simulink model "HeadlightManagement_Test_Harness"  (R2024a)
settings: Solver=FixedStepDiscrete  StartTime=0.0  StopTime=Inf  FixedStep=0.2  RelTol=1e-3  EnableMultiTasking=on
values from neighbouring files (symbols this model uses):
  Dem_EventStatusType : value not decoded    [dict.sldd]
undefined symbols (not defined in the file or in its folder): D1, P
libraries: simulink x6, autosarlibdem x2, autosarlibnvm x1
(part 2 of 2)

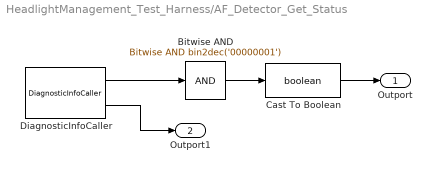
== system HeadlightManagement_Test_Harness/AF_Detector_Get_Status ==
  Bitwise AND : simulink/Logic and Bit Operations/Bitwise Operator  logicop=AND  UseBitMask=on  BitMask=bin2dec('00000001')  BitMaskRealWorld=Stored Integer
      settings: LibrarySourceBlock=|
      | simulink/Quick Insert/Logic and Bit
      | Operations/Bitwise AND
  Cast To Boolean : DataTypeConversion  OutDataTypeStr=boolean  SaturateOnIntegerOverflow=off  RndMeth=Floor
  DiagnosticInfoCaller : autosarlibdem/DiagnosticInfoCaller  PortName=AF_Detector  Operation=GetEventStatus  st=2  ServiceImpl=autosar.bsw.DemDiagnosticInfo  SyncToSchema=off
  Outport : Outport
  Outport1 : Outport  Port=2
  wires:
  Bitwise AND/1 -> Cast To Boolean/1
  Cast To Boolean/1 -> Outport/1
  DiagnosticInfoCaller/1 -> Bitwise AND/1
  DiagnosticInfoCaller/2 -> Outport1/1

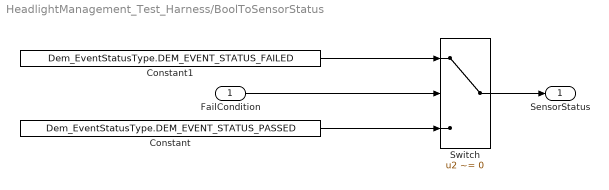
== system HeadlightManagement_Test_Harness/BoolToSensorStatus ==
  FailCondition : Inport
  Constant : Constant  Value=Dem_EventStatusType.DEM_EVENT_STATUS_PASSED
  Constant1 : Constant  Value=Dem_EventStatusType.DEM_EVENT_STATUS_FAILED
  Switch : Switch  Criteria=u2 ~= 0  SaturateOnIntegerOverflow=off  InputSameDT=off
  SensorStatus : Outport  VectorParamsAs1DForOutWhenUnconnected=off
  wires:
  FailCondition/1 -> Switch/2
  Constant/1 -> Switch/3
  Constant1/1 -> Switch/1
  Switch/1 -> SensorStatus/1

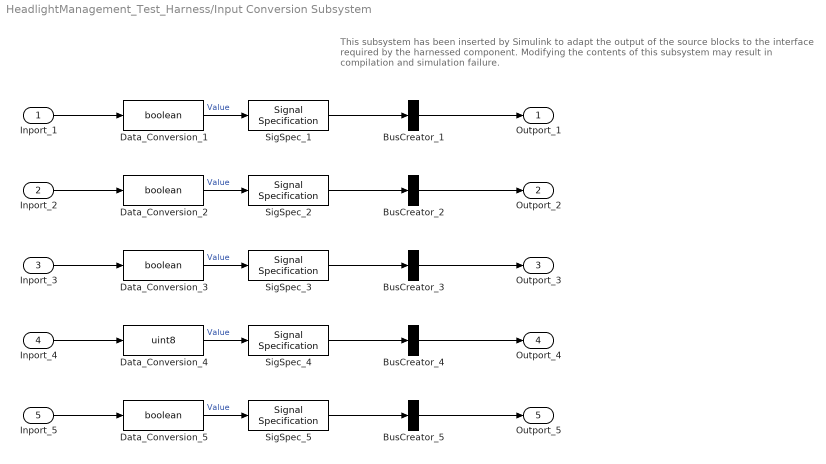
== system HeadlightManagement_Test_Harness/Input Conversion Subsystem ==
  note: This subsystem has been inserted by Simulink to adapt the output of the source blocks to the interface required by the harnessed component.
      |  Modifying the contents of this subsystem may result in compilation and simulation failure.
  Inport_1 : Inport
  Inport_2 : Inport  Port=2
  Inport_3 : Inport  Port=3
  Inport_4 : Inport  Port=4
  Inport_5 : Inport  Port=5
  BusCreator_1 : BusCreator  Inputs=1  OutDataTypeStr=Bus: Sensor_to_Ctrl
  BusCreator_2 : BusCreator  Inputs=1  OutDataTypeStr=Bus: Sensor_to_Ctrl
  BusCreator_3 : BusCreator  Inputs=1  OutDataTypeStr=Bus: HighBeam_Cmd
  BusCreator_4 : BusCreator  Inputs=1  OutDataTypeStr=Bus: TurnSignal_Cmd
  BusCreator_5 : BusCreator  Inputs=1  OutDataTypeStr=Bus: Ignition_State
  Data_Conversion_{1..3,5} (4 alike) : DataTypeConversion  OutDataTypeStr=boolean
  Data_Conversion_4 : DataTypeConversion  OutDataTypeStr=uint8
  SigSpec_1 : SignalSpecification  OutDataTypeStr=boolean  Dimensions=[1]  SampleTime=[-1, 0]
  SigSpec_2 : SignalSpecification  OutDataTypeStr=boolean  Dimensions=[1]  SampleTime=[-1, 0]
  SigSpec_3 : SignalSpecification  OutDataTypeStr=boolean  Dimensions=[1]  SampleTime=0.2
  SigSpec_4 : SignalSpecification  OutDataTypeStr=uint8  Dimensions=[1]  SampleTime=0.2
  SigSpec_5 : SignalSpecification  OutDataTypeStr=boolean  Dimensions=[1]  SampleTime=[-1, 0]
  Outport_1 : Outport
  Outport_2 : Outport  Port=2
  Outport_3 : Outport  Port=3
  Outport_4 : Outport  Port=4
  Outport_5 : Outport  Port=5
  wires:
  BusCreator_1/1 -> Outport_1/1
  SigSpec_1/1 -> BusCreator_1/1
  Data_Conversion_1/1 -> SigSpec_1/1  "Value"
  Inport_1/1 -> Data_Conversion_1/1
  BusCreator_2/1 -> Outport_2/1
  SigSpec_2/1 -> BusCreator_2/1
  Data_Conversion_2/1 -> SigSpec_2/1  "Value"
  Inport_2/1 -> Data_Conversion_2/1
  BusCreator_3/1 -> Outport_3/1
  SigSpec_3/1 -> BusCreator_3/1
  Data_Conversion_3/1 -> SigSpec_3/1  "Value"
  Inport_3/1 -> Data_Conversion_3/1
  BusCreator_4/1 -> Outport_4/1
  SigSpec_4/1 -> BusCreator_4/1
  Data_Conversion_4/1 -> SigSpec_4/1  "Value"
  Inport_4/1 -> Data_Conversion_4/1
  BusCreator_5/1 -> Outport_5/1
  SigSpec_5/1 -> BusCreator_5/1
  Data_Conversion_5/1 -> SigSpec_5/1  "Value"
  Inport_5/1 -> Data_Conversion_5/1

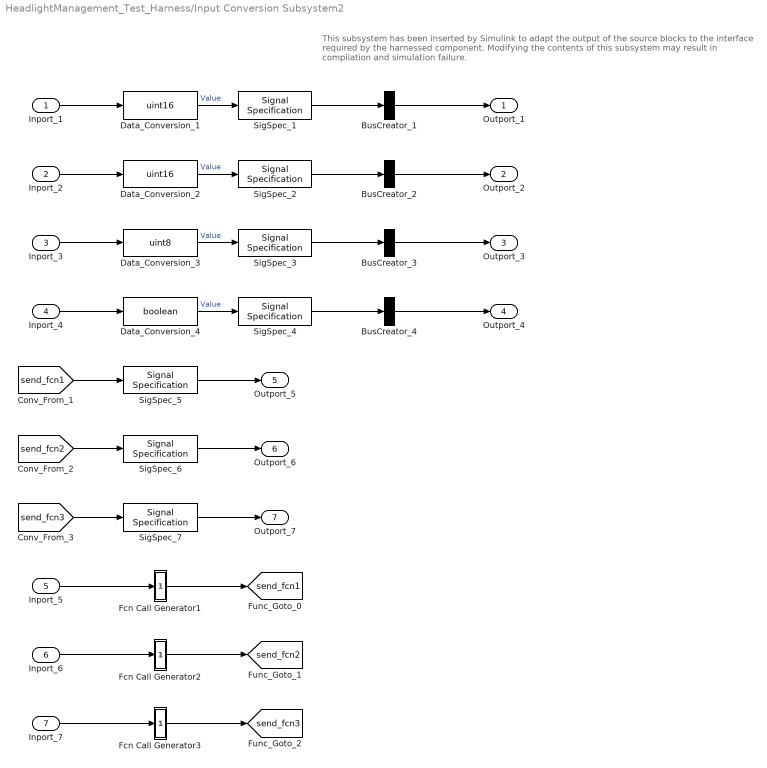
== system HeadlightManagement_Test_Harness/Input Conversion Subsystem2 ==
  note: This subsystem has been inserted by Simulink to adapt the output of the source blocks to the interface required by the harnessed component.
      |  Modifying the contents of this subsystem may result in compilation and simulation failure.
  Inport_1 : Inport
  Inport_2 : Inport  Port=2
  Inport_3 : Inport  Port=3
  Inport_4 : Inport  Port=4
  Inport_5 : Inport  Port=5
  Inport_6 : Inport  Port=6
  Inport_7 : Inport  Port=7
  BusCreator_1 : BusCreator  Inputs=1  OutDataTypeStr=Bus: Light_Data
  BusCreator_2 : BusCreator  Inputs=1  OutDataTypeStr=Bus: Visibility_Distance
  BusCreator_3 : BusCreator  Inputs=1  OutDataTypeStr=Bus: Humidity_Data
  BusCreator_4 : BusCreator  Inputs=1  OutDataTypeStr=Bus: Ignition_State
  Data_Conversion_1 : DataTypeConversion  OutDataTypeStr=uint16
  Data_Conversion_2 : DataTypeConversion  OutDataTypeStr=uint16
  Data_Conversion_3 : DataTypeConversion  OutDataTypeStr=uint8
  Data_Conversion_4 : DataTypeConversion  OutDataTypeStr=boolean
  Fcn Call Generator1 : Subsystem  Tag=_SLT_FCN_CALL_GEN_BLK_  mask(Function Call Generator Subsystem){sample_time=-1}
      mask prompts: sample_time "Sample time:"
      settings: LibrarySourceBlock=sltestutillib/fcn_call_gen
  Fcn Call Generator2 : Subsystem  Tag=_SLT_FCN_CALL_GEN_BLK_  mask(Function Call Generator Subsystem){sample_time=-1}
      mask prompts: sample_time "Sample time:"
      settings: LibrarySourceBlock=sltestutillib/fcn_call_gen
  Fcn Call Generator3 : Subsystem  Tag=_SLT_FCN_CALL_GEN_BLK_  mask(Function Call Generator Subsystem){sample_time=-1}
      mask prompts: sample_time "Sample time:"
      settings: LibrarySourceBlock=sltestutillib/fcn_call_gen
  SigSpec_1 : SignalSpecification  OutDataTypeStr=uint16  Unit=lx  Dimensions=[1]
  SigSpec_2 : SignalSpecification  OutDataTypeStr=uint16  Unit=meter  Dimensions=[1]
  SigSpec_3 : SignalSpecification  OutDataTypeStr=uint8  Unit=%RH  Dimensions=[1]
  SigSpec_4 : SignalSpecification  OutDataTypeStr=boolean  Dimensions=[1]
  SigSpec_5 : SignalSpecification
  SigSpec_6 : SignalSpecification
  SigSpec_7 : SignalSpecification
  Outport_1 : Outport
  Outport_2 : Outport  Port=2
  Outport_3 : Outport  Port=3
  Outport_4 : Outport  Port=4
  Outport_5 : Outport  Port=5
  Outport_6 : Outport  Port=6
  Outport_7 : Outport  Port=7
  tag scope: send_fcn1=global, send_fcn2=global, send_fcn3=global
  wires:
  BusCreator_1/1 -> Outport_1/1
  SigSpec_1/1 -> BusCreator_1/1
  Data_Conversion_1/1 -> SigSpec_1/1  "Value"
  Inport_1/1 -> Data_Conversion_1/1
  BusCreator_2/1 -> Outport_2/1
  SigSpec_2/1 -> BusCreator_2/1
  Data_Conversion_2/1 -> SigSpec_2/1  "Value"
  Inport_2/1 -> Data_Conversion_2/1
  BusCreator_3/1 -> Outport_3/1
  SigSpec_3/1 -> BusCreator_3/1
  Data_Conversion_3/1 -> SigSpec_3/1  "Value"
  Inport_3/1 -> Data_Conversion_3/1
  BusCreator_4/1 -> Outport_4/1
  SigSpec_4/1 -> BusCreator_4/1
  Data_Conversion_4/1 -> SigSpec_4/1  "Value"
  Inport_4/1 -> Data_Conversion_4/1
  SigSpec_5/1 -> Outport_5/1
  [send_fcn1] -> SigSpec_5/1
  SigSpec_6/1 -> Outport_6/1
  [send_fcn2] -> SigSpec_6/1
  SigSpec_7/1 -> Outport_7/1
  [send_fcn3] -> SigSpec_7/1
  Fcn Call Generator1/1(Out1) -> [send_fcn1]
  Inport_5/1 -> Fcn Call Generator1/1(In1)
  Fcn Call Generator2/1(Out1) -> [send_fcn2]
  Inport_6/1 -> Fcn Call Generator2/1(In1)
  Fcn Call Generator3/1(Out1) -> [send_fcn3]
  Inport_7/1 -> Fcn Call Generator3/1(In1)

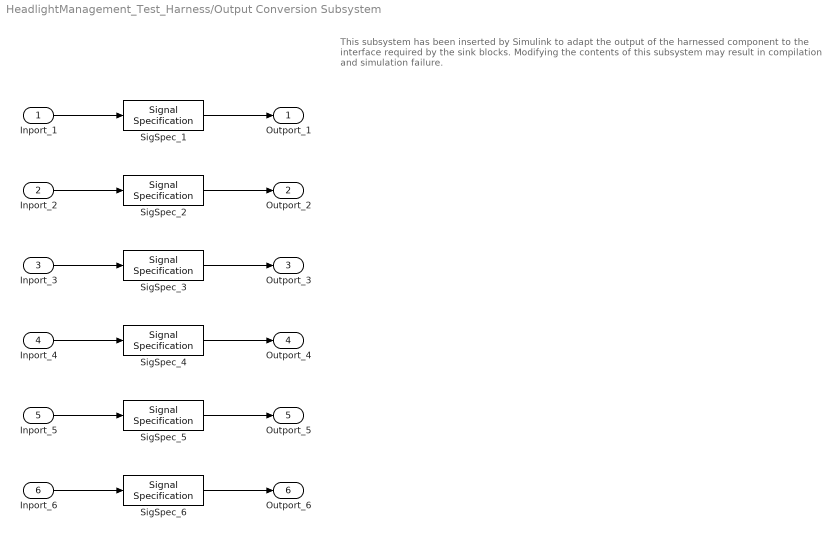
== system HeadlightManagement_Test_Harness/Output Conversion Subsystem ==
  note: This subsystem has been inserted by Simulink to adapt the output of the harnessed component to the interface required by the sink blocks.
      |  Modifying the contents of this subsystem may result in compilation and simulation failure.
  Inport_1 : Inport
  Inport_2 : Inport  Port=2
  Inport_3 : Inport  Port=3
  Inport_4 : Inport  Port=4
  Inport_5 : Inport  Port=5
  Inport_6 : Inport  Port=6
  SigSpec_{1..6} (6 alike) : SignalSpecification  Dimensions=[-1]  SampleTime=0.2
  Outport_1 : Outport
  Outport_2 : Outport  Port=2
  Outport_3 : Outport  Port=3
  Outport_4 : Outport  Port=4
  Outport_5 : Outport  Port=5
  Outport_6 : Outport  Port=6
  wires:
  Inport_1/1 -> SigSpec_1/1
  SigSpec_1/1 -> Outport_1/1
  Inport_2/1 -> SigSpec_2/1
  SigSpec_2/1 -> Outport_2/1
  Inport_3/1 -> SigSpec_3/1
  SigSpec_3/1 -> Outport_3/1
  Inport_4/1 -> SigSpec_4/1
  SigSpec_4/1 -> Outport_4/1
  Inport_5/1 -> SigSpec_5/1
  SigSpec_5/1 -> Outport_5/1
  Inport_6/1 -> SigSpec_6/1
  SigSpec_6/1 -> Outport_6/1

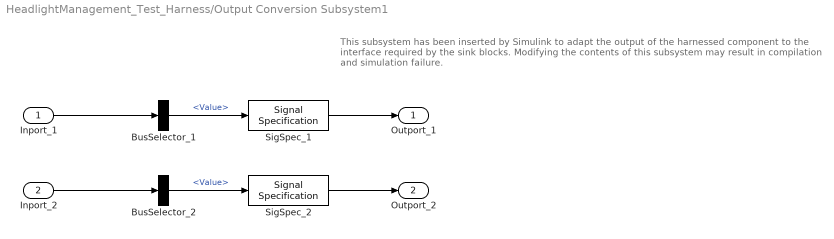
== system HeadlightManagement_Test_Harness/Output Conversion Subsystem1 ==
  note: This subsystem has been inserted by Simulink to adapt the output of the harnessed component to the interface required by the sink blocks.
      |  Modifying the contents of this subsystem may result in compilation and simulation failure.
  Inport_1 : Inport
  Inport_2 : Inport  Port=2
  BusSelector_1 : BusSelector  OutputSignals=Value
  BusSelector_2 : BusSelector  OutputSignals=Value
  SigSpec_1 : SignalSpecification  OutDataTypeStr=boolean  Dimensions=[1]
  SigSpec_2 : SignalSpecification  OutDataTypeStr=boolean  Dimensions=[1]
  Outport_1 : Outport
  Outport_2 : Outport  Port=2
  wires:
  Inport_1/1 -> BusSelector_1/1
  BusSelector_1/1 -> SigSpec_1/1  "<Value>"
  SigSpec_1/1 -> Outport_1/1
  Inport_2/1 -> BusSelector_2/1
  BusSelector_2/1 -> SigSpec_2/1  "<Value>"
  SigSpec_2/1 -> Outport_2/1

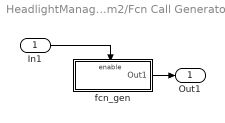
== system HeadlightManagement_Test_Harness/Input Conversion Subsystem2/Fcn Call Generator1 ==
  In1 : Inport  OutDataTypeStr=boolean
  fcn_gen : Subsystem  TreatAsAtomicUnit=on
  Out1 : Outport  VectorParamsAs1DForOutWhenUnconnected=off
  wires:
  fcn_gen/1(Out1) -> Out1/1
  In1/1 -> fcn_gen/Enable

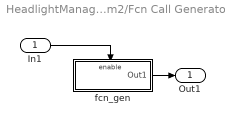
== system HeadlightManagement_Test_Harness/Input Conversion Subsystem2/Fcn Call Generator2 ==
  In1 : Inport  OutDataTypeStr=boolean
  fcn_gen : Subsystem  TreatAsAtomicUnit=on
  Out1 : Outport  VectorParamsAs1DForOutWhenUnconnected=off
  wires:
  fcn_gen/1(Out1) -> Out1/1
  In1/1 -> fcn_gen/Enable

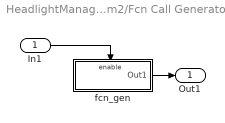
== system HeadlightManagement_Test_Harness/Input Conversion Subsystem2/Fcn Call Generator3 ==
  In1 : Inport  OutDataTypeStr=boolean
  fcn_gen : Subsystem  TreatAsAtomicUnit=on
  Out1 : Outport  VectorParamsAs1DForOutWhenUnconnected=off
  wires:
  fcn_gen/1(Out1) -> Out1/1
  In1/1 -> fcn_gen/Enable

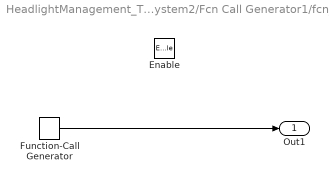
== system HeadlightManagement_Test_Harness/Input Conversion Subsystem2/Fcn Call Generator1/fcn_gen ==
  Enable : EnablePort
  Function-Call Generator : simulink/Ports & Subsystems/Function-Call Generator  sample_time=sample_time  numberOfIterations=1  DisallowWideOutput=off
  Out1 : Outport  VectorParamsAs1DForOutWhenUnconnected=off
  wires:
  Function-Call Generator/1 -> Out1/1

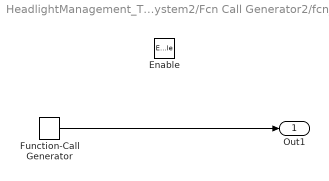
== system HeadlightManagement_Test_Harness/Input Conversion Subsystem2/Fcn Call Generator2/fcn_gen ==
  Enable : EnablePort
  Function-Call Generator : simulink/Ports & Subsystems/Function-Call Generator  sample_time=sample_time  numberOfIterations=1  DisallowWideOutput=off
  Out1 : Outport  VectorParamsAs1DForOutWhenUnconnected=off
  wires:
  Function-Call Generator/1 -> Out1/1

== system HeadlightManagement_Test_Harness/Input Conversion Subsystem2/Fcn Call Generator3/fcn_gen ==
  Enable : EnablePort
  Function-Call Generator : simulink/Ports & Subsystems/Function-Call Generator  sample_time=sample_time  numberOfIterations=1  DisallowWideOutput=off
  Out1 : Outport  VectorParamsAs1DForOutWhenUnconnected=off
  wires:
  Function-Call Generator/1 -> Out1/1
